simulink subsystem "bare_trans_QPSK"  (R2024b)
settings: Solver=VariableStepAuto  StartTime=0.0  StopTime=10.0  RelTol=1e-3
undefined symbols (not defined in the file or in its folder): Param
libraries: commfilt2 x1, commdigbbndpm3 x1
settings Model: Creator=rober  LastModifiedBy=rober

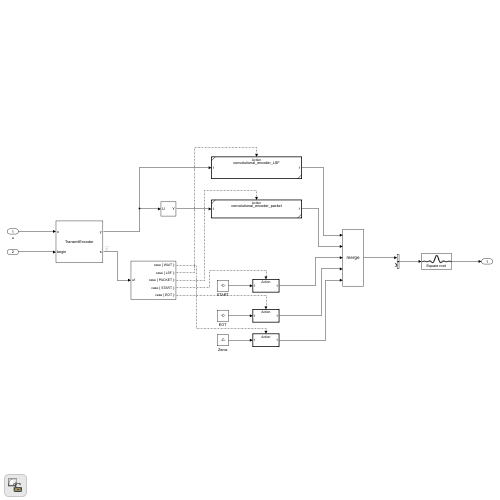
[thumbnail: Simulink's stored preview of the top-level diagram]
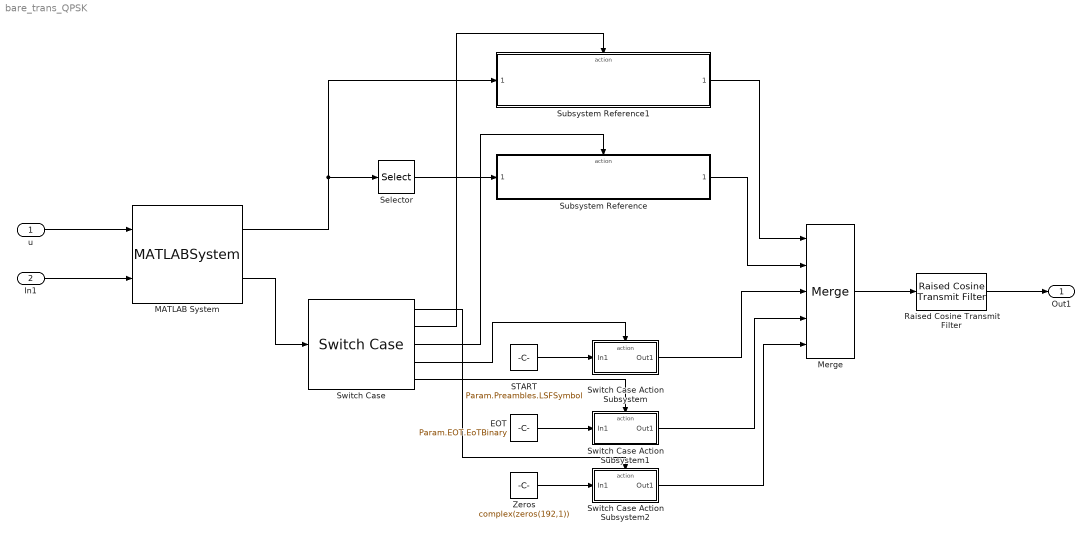
== system bare_trans_QPSK ==
  u : Inport
  In1 : Inport  Port=2
  EOT : Constant  Value=Param.EOT.EoTBinary  VectorParams1D=off
  MATLAB System : MATLABSystem  System=TransmitEncoder  Source=Param.Source  Destination=Param.Destination  FrameLength=240  SimulateUsing=Code generation
      mask Type: TransmitEncoder
      mask Display:
      | disp('TransmitEncoder');
      | port_label('input',1,'x');
      | port_label('input',2,'begin');
      | port_label('output',1,'y');
      | port_label('output',2,'s');
  Merge : Merge  Inputs=5
  Raised Cosine Transmit Filter : commfilt2/Raised Cosine Transmit Filter  filtType=Square root  R=Param.RolloffFactor  filtSpan=Param.RaisedCosineFilterSpan  N=Param.Interpolation  filterGain=1/4  InputProcessing=Columns as channels (frame based)  RateOptions=Enforce single-rate processing  framing=Mute  checkCoeff=off  variableName=rcTxFilt  checkGain=Normalized  sampMode=Mute  saveAsFlag=0  currentFiltSpan=10  D=(10)/2  launchFVT=on  roundingMode=Floor  overflowMode=off  coeffDataTypeStr=Inherit: Same word length as input  coeffMin=[]  coeffMax=[]  coeffLastDataTypeStr=Inherit: Same word length as input  outputDataTypeStr=Inherit: Same as accumulator  outputMin=[]  outputMax=[]  outputLastDataTypeStr=Inherit: Same as accumulator
  START : Constant  Value=Param.Preambles.LSFSymbol  VectorParams1D=off
  Selector : Selector  IndexOptions=Index vector (dialog)  Indices=[1:206]  OutputSizes=1
  Subsystem Reference : Subsystem  ReferencedSubsystem=convolutional_encoder_packet
  Subsystem Reference1 : Subsystem  ReferencedSubsystem=convolutional_encoder_LSF
  Switch Case : SwitchCase  CaseConditions={transmitEncoderStates.WAIT,transmitEncoderStates.LSF, transmitEncoderStates.PACKET, transmitEncoderStates.START, transmitEncoderStates.EOT}  ShowDefaultCase=off
  Switch Case Action Subsystem : Subsystem  TreatAsAtomicUnit=on
  Switch Case Action Subsystem1 : Subsystem  TreatAsAtomicUnit=on
  Switch Case Action Subsystem2 : Subsystem  TreatAsAtomicUnit=on
  Zeros : Constant  Value=complex(zeros(192,1))  VectorParams1D=off
  Out1 : Outport
  wires:
  Raised Cosine Transmit Filter/1 -> Out1/1
  u/1 -> MATLAB System/1
  In1/1 -> MATLAB System/2
  MATLAB System/2 -> Switch Case/1
  Subsystem Reference1/1 -> Merge/1
  Subsystem Reference/1 -> Merge/2
  MATLAB System/1 -> Subsystem Reference1/1, Selector/1
  Selector/1 -> Subsystem Reference/1
  EOT/1 -> Switch Case Action Subsystem1/1(In1)
  Switch Case Action Subsystem1/1(Out1) -> Merge/4
  START/1 -> Switch Case Action Subsystem/1(In1)
  Switch Case Action Subsystem/1(Out1) -> Merge/3
  Zeros/1 -> Switch Case Action Subsystem2/1(In1)
  Switch Case Action Subsystem2/1(Out1) -> Merge/5
  Switch Case/1 -> Switch Case Action Subsystem2/Action
  Switch Case/2 -> Subsystem Reference1/Action
  Switch Case/3 -> Subsystem Reference/Action
  Switch Case/4 -> Switch Case Action Subsystem/Action
  Switch Case/5 -> Switch Case Action Subsystem1/Action
  Merge/1 -> Raised Cosine Transmit Filter/1

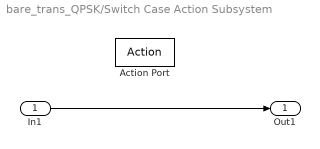
== system bare_trans_QPSK/Switch Case Action Subsystem ==
  In1 : Inport
  Action Port : ActionPort
  Out1 : Outport
  wires:
  In1/1 -> Out1/1

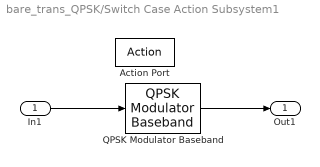
== system bare_trans_QPSK/Switch Case Action Subsystem1 ==
  In1 : Inport
  Action Port : ActionPort
  QPSK Modulator Baseband : commdigbbndpm3/QPSK Modulator Baseband  InType=Bit  Enc=Binary  Ph=pi/4  outDtype=double  outWordLen=16  outUDDataType=sfix(16)  outFracLenMode=Best precision  outFracLen=15  outDataTypeStr=double  outLastDataTypeStr=double
  Out1 : Outport
  wires:
  QPSK Modulator Baseband/1 -> Out1/1
  In1/1 -> QPSK Modulator Baseband/1

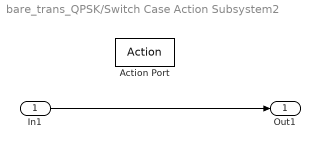
== system bare_trans_QPSK/Switch Case Action Subsystem2 ==
  In1 : Inport
  Action Port : ActionPort
  Out1 : Outport
  wires:
  In1/1 -> Out1/1
